simulink model "ms_thesis_trajectory"  (R2023a)
settings: Solver=VariableStepAuto  StartTime=0.0  StopTime=10.0  RelTol=1e-3
undefined symbols (not defined in the file): Aircraft
libraries: simulink x2
settings Model: Creator=redro  LastModifiedBy=redro

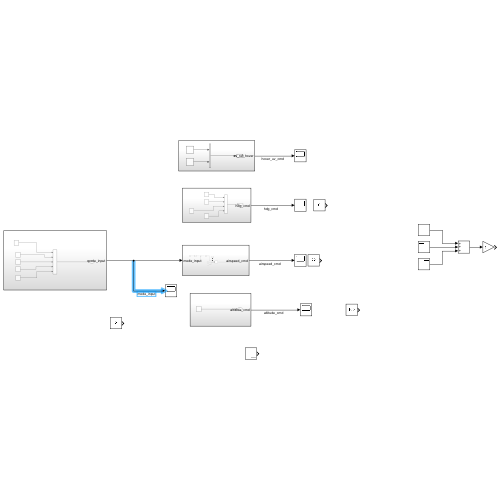
[thumbnail: Simulink's stored preview of the top-level diagram]
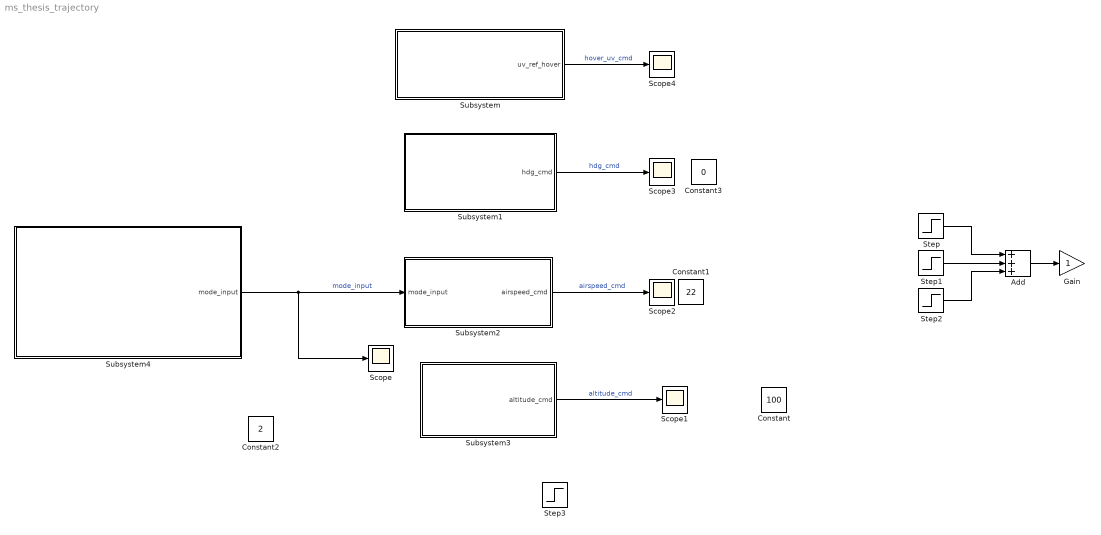
== system ms_thesis_trajectory ==
  Add : Sum  Inputs=+++
  Constant : Constant  Value=100  OutDataTypeStr=single
  Constant1 : Constant  Value=22  OutDataTypeStr=single
  Constant2 : Constant  Value=2  OutDataTypeStr=single
  Constant3 : Constant  Value=0  OutDataTypeStr=single
  Gain : Gain
  Scope{,1..4} (5 alike) : Scope
  Step : Step  Time=6  OutDataTypeStr=single  SampleTime=0
  Step1 : Step  Time=12  Before=1  After=-1  OutDataTypeStr=single  SampleTime=0
  Step2 : Step  Time=18  Before=-1  After=0  OutDataTypeStr=single  SampleTime=0
  Step3 : Step  Time=3  Before=100  After=90  OutDataTypeStr=single  SampleTime=0
  Subsystem : Subsystem
  Subsystem1 : Subsystem
  Subsystem2 : Subsystem
  Subsystem3 : Subsystem
  Subsystem4 : Subsystem
  wires:
  Add/1 -> Gain/1
  Step/1 -> Add/1
  Step1/1 -> Add/2
  Subsystem/1(uv_ref_hover) -> Scope4/1  "hover_uv_cmd"
  Step2/1 -> Add/3
  Subsystem2/1(airspeed_cmd) -> Scope2/1  "airspeed_cmd"
  Subsystem1/1(hdg_cmd) -> Scope3/1  "hdg_cmd"
  Subsystem4/1(mode_input) -> Scope/1, Subsystem2/1(mode_input)  "mode_input"
  Subsystem3/1(altitude_cmd) -> Scope1/1  "altitude_cmd"

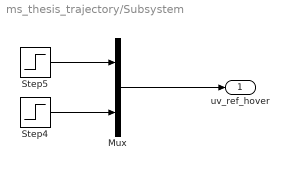
== system ms_thesis_trajectory/Subsystem ==
  Mux : Mux  Inputs=2
  Step4 : Step  Time=73  After=3  OutDataTypeStr=single  SampleTime=0
  Step5 : Step  Time=27  After=0  OutDataTypeStr=single  SampleTime=0
  uv_ref_hover : Outport
  wires:
  Step5/1 -> Mux/1
  Mux/1 -> uv_ref_hover/1
  Step4/1 -> Mux/2

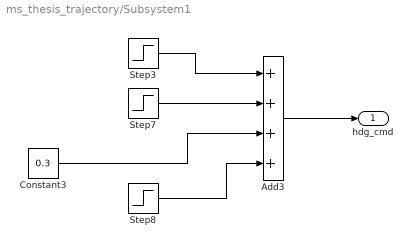
== system ms_thesis_trajectory/Subsystem1 ==
  Add3 : Sum  Inputs=++++
  Constant3 : Constant  Value=0.3  OutDataTypeStr=single
  Step3 : Step  Time=2  After=-0.8  OutDataTypeStr=single  SampleTime=0
  Step7 : Step  Time=18  Before=-0.8  After=0.5  OutDataTypeStr=single  SampleTime=0
  Step8 : Step  Time=30  Before=0.5  After=2.75  OutDataTypeStr=single  SampleTime=0
  hdg_cmd : Outport
  wires:
  Step7/1 -> Add3/2
  Step8/1 -> Add3/4
  Constant3/1 -> Add3/3
  Add3/1 -> hdg_cmd/1
  Step3/1 -> Add3/1

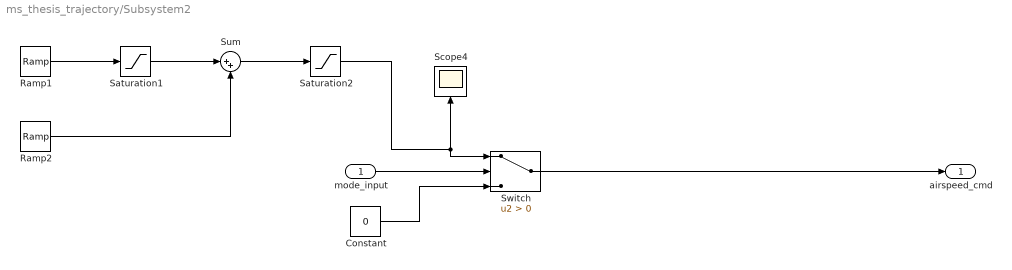
== system ms_thesis_trajectory/Subsystem2 ==
  mode_input : Inport
  Constant : Constant  Value=0  OutDataTypeStr=single
  Ramp1 : simulink/Sources/Ramp  slope=Aircraft.Control.modes.hover2forward_airspeed_ramp  start=7  InitialOutput=0
  Ramp2 : simulink/Sources/Ramp  slope=Aircraft.Control.modes.forward2hover_airspeed_ramp  start=52  InitialOutput=0
  Saturation1 : Saturate  UpperLimit=22  LowerLimit=0  OutDataTypeStr=single
  Saturation2 : Saturate  UpperLimit=22  LowerLimit=0  OutDataTypeStr=single
  Scope4 : Scope
  Sum : Sum  Inputs=|++
  Switch : Switch  Criteria=u2 > Threshold  SaturateOnIntegerOverflow=off  InputSameDT=off
  airspeed_cmd : Outport
  wires:
  Ramp1/1 -> Saturation1/1
  Constant/1 -> Switch/3
  Ramp2/1 -> Sum/2
  Saturation2/1 -> Switch/1, Scope4/1
  Sum/1 -> Saturation2/1
  Saturation1/1 -> Sum/1
  mode_input/1 -> Switch/2
  Switch/1 -> airspeed_cmd/1

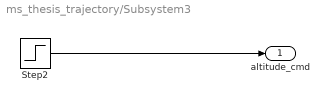
== system ms_thesis_trajectory/Subsystem3 ==
  Step2 : Step  Time=48  Before=100  After=90  OutDataTypeStr=single  SampleTime=0
  altitude_cmd : Outport
  wires:
  Step2/1 -> altitude_cmd/1

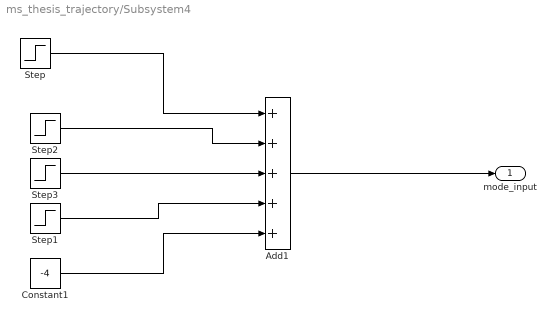
== system ms_thesis_trajectory/Subsystem4 ==
  Add1 : Sum  Inputs=+++++
  Constant1 : Constant  Value=-4
  Step : Step  Time=7  SampleTime=0
  Step1 : Step  Time=18  Before=1  After=2  SampleTime=0
  Step2 : Step  Time=52  Before=2  SampleTime=0
  Step3 : Step  Time=70  Before=1  After=0  SampleTime=0
  mode_input : Outport
  wires:
  Step2/1 -> Add1/2
  Constant1/1 -> Add1/5
  Step1/1 -> Add1/4
  Step3/1 -> Add1/3
  Step/1 -> Add1/1
  Add1/1 -> mode_input/1
